simulink model "generate_cartesian_velocity_motion"  (R2019a)
settings: Solver=FixedStepDiscrete  StartTime=0.0  StopTime=inf  FixedStep=0.001  RelTol=1e-3  EnableMultiTasking=on
PreLoadFcn:
  | set_param(gcs, 'RTWSystemTargetFile', 'franka_emika_panda.tlc');
  | demos_common_configs();
  | 
  | collision_behavior = ...
  |             [25.0, 25.0, 22.0, 20.0, 19.0, 17.0, 14.0,... % lower_torque_thresholds_acceleration
  |              35.0, 35.0, 32.0, 30.0, 29.0, 27.0, 24.0,... % upper_torque_thresholds_acceleration
  |              25.0, 25.0, 22.0, 20.0, 19.0, 17.0, 14.0,... % lower_torque_thresholds_nominal
  |              35.0, 35.0, 32.0, 30.0, 29.0, 27.0, 24.0,... % upper_torque_thresholds_nominal
  |              30.0, 30.0, 30.0, 25.0, 25.0, 25.0,...       % lower_force_thresholds_acceleration
  |              40.0, 40.0, 40.0, 35.0, 35.0, 35.0,...       % upper_force_thresholds_acceleration
  |              30.0, 30.0, 30.0, 25.0, 25.0, 25.0,...       % lower_force_thresholds_nominal
  |              40.0, 40.0, 40.0, 35.0, 35.0, 35.0];         % upper_force_thresholds_nominal
libraries: simulink x3, franka_simulink_library x2
settings Model: SimulationMode=external  ExtModeTrigDuration=10000  Creator=vasi_ko  LastModifiedBy=konstantinosvasios
settings DataIOCC: LimitDataPoints=on  SaveFormat=Array  ReturnWorkspaceOutputs=off
settings OptimizationCC: DefaultParameterBehavior=Inlined  EnhancedBackFolding=on  PassReuseOutputArgsThreshold=0  OptimizeBlockOrder=speed  DifferentSizesBufferReuse=on  OptimizationCustomize=off
settings DebuggingCC: SolverPrmCheckMsg=warning  ParameterTunabilityLossMsg=error  SFUnexpectedBacktrackingDiag=warning  SFNoUnconditionalDefaultTransitionDiag=warning  SFExecutionAtInitializationDiag=none  ArithmeticOperatorsInVariantConditions=warning
settings HardwareCC: ProdBitPerLong=64  ProdHWDeviceType=Intel->x86-64 (Linux 64)
settings ModelReferenceCC: PropagateSignalLabelsOutOfModel=off
settings SFSimCC: SimUseLocalCustomCode=off  MATLABDynamicMemAlloc=off
settings RTWCC: Description=Generic Real-Time Target  SystemTargetFile=franka_emika_panda.tlc  RTWVerbose=off  RTWUseLocalCustomCode=off  Toolchain=Franka Simulink | gmake (64-bit linux)  BuildConfiguration=Faster Runs  TargetLang=C++
settings CodeAppCC: ForceParamTrailComments=on  OperatorAnnotations=on
settings STFCustomTargetCC: TargetLangStandard=C99 (ISO)  ModelReferenceCompliant=off  MatFileLogging=on  UseToolchainInfoCompliant=on  SystemTargetFile=franka_emika_panda.tlc
settings GRTTargetCC: ModelReferenceCompliant=off  ParMdlRefBuildCompliant=off  CompOptLevelCompliant=off  ConcurrentExecutionCompliant=off  CombineOutputUpdateFcns=off  CPPClassGenCompliant=off  GRTInterface=on  ExtModeTransport=1
settings ConfigComp: CovMetricSettings=dw  CovSaveCumulativeToWorkspaceVar=on  CovSaveSingleToWorkspaceVar=on  CovExternalEMLEnable=off  CovSFcnEnable=off

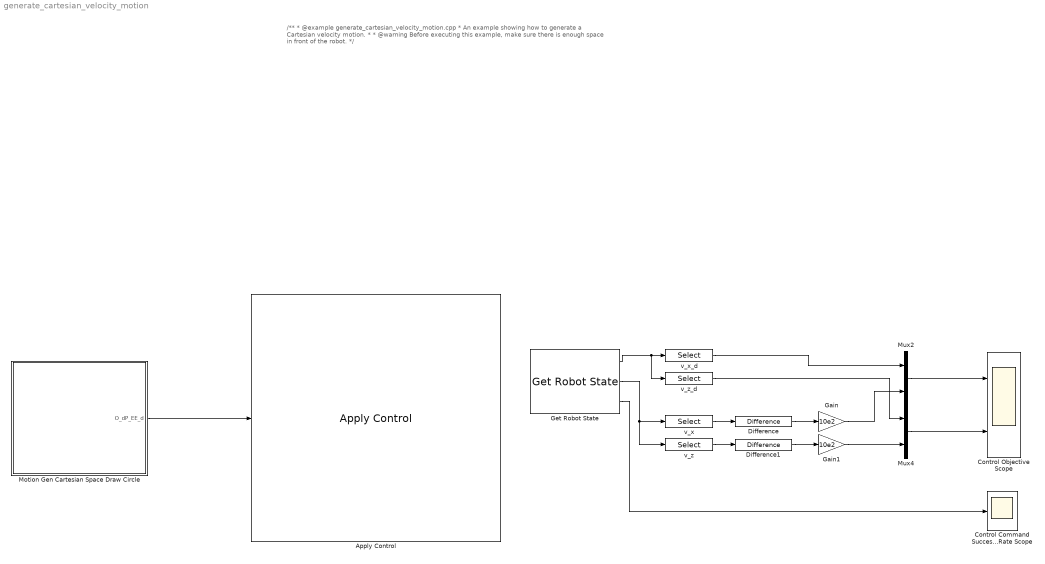
== system generate_cartesian_velocity_motion ==
  note: /**
      |  * @example generate_cartesian_velocity_motion.cpp
      |  * An example showing how to generate a Cartesian velocity motion.
      |  *
      |  * @warning Before executing this example, make sure there is enough space in front of the robot.
      |  */
  Apply Control : franka_simulink_library/Apply Control  robot_ip=robot_ip  gripper_attached=off  control_mode=Cartesian Velocities - Internal Controller Mode  controller_choice=Joint Impedance Controller  elbow_control=off  collision_thresholds=[25.0, 25.0, 22.0, 20.0, 19.0, 17.0, 14.0,35.0, 35.0, 32.0, 30.0, 29.0, 27.0, 24.0,25.0, 25.0, 22.0, 20.0, 19.0, 17.0, 14.0,35.0, 35.0, 32.0, 30.0, 29.0, 27.0, 24.0,30.0, 30.0, 30.0, 25.0, 25.0, 25.0,40.0, 40.0, 40.0, 35.0, 35.0, 35.0,30.0, 30.0, 30.0, 25.0, 25.0, 25.0,40.0, 40.0, 40.0, 35.0, 35.0, 35.0]  joint_impedance=[3000, 3000, 3000, 2500, 2500, 2000, 2000]  cartesian_impedance=cartesian_impedance  load_inertia=load_inertia  EE_T_K=EE_T_K  init_joint_configuration_req=on  init_joint_configuration=q_init
      settings: SourceProductName=Franka Emika
  Control Command Success Rate Scope : Scope
  Control Objective Scope : Scope  NumInputPorts=2
  Difference : simulink/Discrete/Difference  ICPrevInput=0.3069  OutMin=[]  OutMax=[]  OutDataType=fixdt(1, 16)  OutScaling=2^-10  DoSatur=off
  Difference1 : simulink/Discrete/Difference  ICPrevInput=0.5902  OutMin=[]  OutMax=[]  OutDataType=fixdt(1, 16)  OutScaling=2^-10  DoSatur=off
  Gain : Gain  Gain=10e2
  Gain1 : Gain  Gain=10e2
  Get Robot State : franka_simulink_library/Get Robot State  robot_ip=robot_ip  signals_requested='O_dP_EE_c O_T_EE control_command_success_rate'
      settings: SourceProductName=Franka Emika
  Motion Gen Cartesian Space Draw Circle : Subsystem
      mask Display:
      | pos = get_param(gcb, 'Position');
      | width = pos(3) - pos(1);
      | x = [0:width];
      | y = sin(x/180*pi);
      | % Parameters 'm' and 'b' must be defined in 'Parameters & Dialog' pane.
      | plot((1/2)*cos(x/180*2*pi+pi/4), (1/2)*sin(x/180*2*pi+pi/4));
      | 
      | port_label('output',1,'O_dP_EE_d');
  Mux2 : Mux  Inputs=2
  Mux4 : Mux  Inputs=2
  v_x : Selector  InputPortWidth=16  IndexOptions=Index vector (dialog)  Indices=13  OutputSizes=1
  v_x_d : Selector  InputPortWidth=6  IndexOptions=Index vector (dialog)  Indices=1  OutputSizes=1
  v_z : Selector  InputPortWidth=16  IndexOptions=Index vector (dialog)  Indices=15  OutputSizes=1
  v_z_d : Selector  InputPortWidth=6  IndexOptions=Index vector (dialog)  Indices=3  OutputSizes=1
  wires:
  Motion Gen Cartesian Space Draw Circle/1(O_dP_EE_d) -> Apply Control/1
  Get Robot State/1 -> v_x_d/1, v_z_d/1
  Get Robot State/2 -> v_z/1, v_x/1
  v_x/1 -> Difference/1
  v_z/1 -> Difference1/1
  Difference/1 -> Gain/1
  Difference1/1 -> Gain1/1
  Gain1/1 -> Mux4/2
  Gain/1 -> Mux2/2
  v_x_d/1 -> Mux2/1
  v_z_d/1 -> Mux4/1
  Mux2/1 -> Control Objective Scope/1
  Mux4/1 -> Control Objective Scope/2
  Get Robot State/3 -> Control Command Success Rate Scope/1

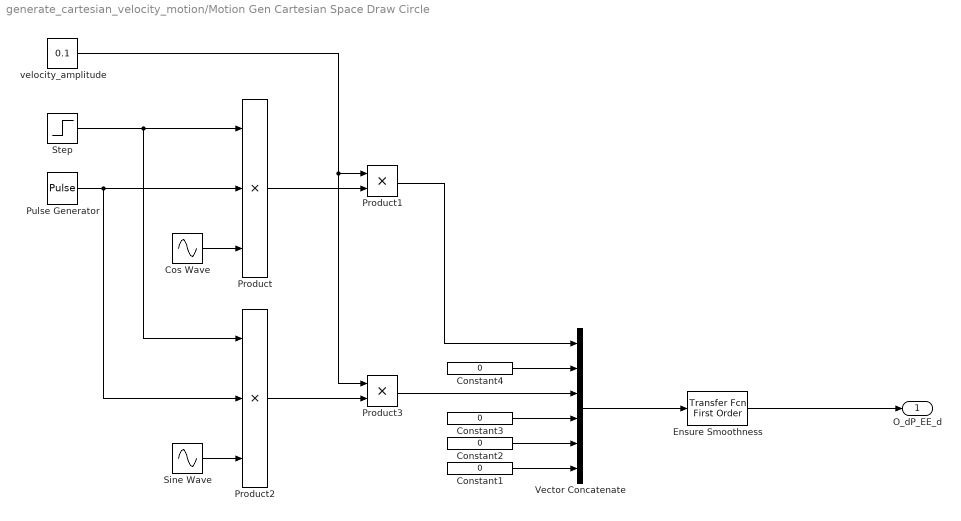
== system generate_cartesian_velocity_motion/Motion Gen Cartesian Space Draw Circle ==
  Constant{1..4} (4 alike) : Constant  Value=0  VectorParams1D=off
  Cos Wave : Sin  Frequency=pi  Phase=pi+pi/2  SampleTime=0
  Ensure Smoothness : simulink/Discrete/Transfer Fcn First Order  PoleZ=0.99  ICPrevOutput=0.0  DoSatur=off
  Product : Product  Inputs=3
  Product1 : Product
  Product2 : Product  Inputs=3
  Product3 : Product
  Pulse Generator : DiscretePulseGenerator  PulseType=Time based  Period=20  PulseWidth=50  PhaseDelay=1
  Sine Wave : Sin  Frequency=pi  Phase=pi  SampleTime=0
  Step : Step  Time=9  Before=1  After=0  SampleTime=0
  Vector Concatenate : Concatenate  NumInputs=6
  velocity_amplitude : Constant  Value=0.1  VectorParams1D=off
  O_dP_EE_d : Outport  VectorParamsAs1DForOutWhenUnconnected=off
  wires:
  Product1/1 -> Vector Concatenate/1
  Product3/1 -> Vector Concatenate/3
  Product2/1 -> Product3/2
  Sine Wave/1 -> Product2/3
  Pulse Generator/1 -> Product/2, Product2/2
  Step/1 -> Product/1, Product2/1
  velocity_amplitude/1 -> Product1/1, Product3/1
  Constant4/1 -> Vector Concatenate/2
  Constant3/1 -> Vector Concatenate/4
  Constant2/1 -> Vector Concatenate/5
  Constant1/1 -> Vector Concatenate/6
  Vector Concatenate/1 -> Ensure Smoothness/1
  Product/1 -> Product1/2
  Cos Wave/1 -> Product/3
  Ensure Smoothness/1 -> O_dP_EE_d/1
